simulink model "GNC_exp"  (R2018a)
settings: Solver=FixedStepAuto  StartTime=0.0  StopTime=50  FixedStep=0.05  MaxStep=0.5  MinStep=0.3  RelTol=10  AbsTol=10
values from neighbouring files (symbols this model uses):
  flightplan = [3.3,0,height,deg2rad(0) ... (first row only)    [initialize_exp.m]
  g = 9.81    [initialize_exp.m]
  HFOV = VFOV*resolution(1)/resolution(2)    [initialize_exp.m]
  max_rot_Z = (13)*pi/180    (= 0.226892802759)    [initialize_exp.m]
  max_theta_X = 8*pi/180    (= 0.13962634016)    [initialize_exp.m]
  max_theta_Y = 8*pi/180    (= 0.13962634016)    [initialize_exp.m]
  max_v_Z = 1*max_vel    (= 0.5)    [initialize_exp.m]
  max_vel = 0.5    [initialize_exp.m]
  spline_init = [P0;P1;P2;P3]    [initialize_exp.m]
  two_std_dev_init = [1,1,0.3,deg2rad(15)]    [initialize_exp.m]
  two_std_dev_thres = 0.2    [initialize_exp.m]
  VFOV = 1.05    [initialize_exp.m]
undefined symbols (not defined in the file or in its folder): eul, pos, vel
libraries: sharedtransform x3, aerolibutil x2, simulink x1
(part 1 of 2)
settings Model: EnablePacing=on  Creator=vinni  LastModifiedBy=lenny
settings SolverCC: MaxConsecutiveMinStep=99999  ShapePreserveControl=EnableAll  ZeroCrossAlgorithm=Adaptive
settings DebuggingCC: WriteAfterWriteMsg=EnableAllAsError  AlgebraicLoopMsg=error  IntegerOverflowMsg=error  ParameterUnderflowMsg=error  UniqueDataStoreMsg=error  NonBusSignalsTreatedAsBus=error  IntegerSaturationMsg=error
settings HardwareCC: ProdBitPerLong=64  ProdHWDeviceType=Intel->x86-64 (Linux 64)

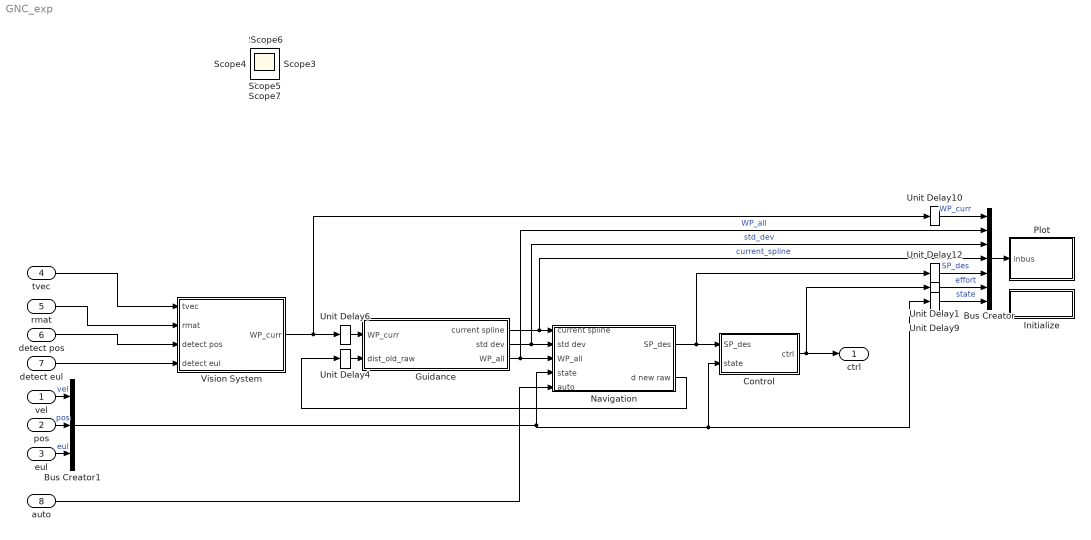
== system GNC_exp ==
  vel : Inport
  pos : Inport  Port=2
  eul : Inport  Port=3
  tvec : Inport  Port=4  PortDimensions=[3,1]
  rmat : Inport  Port=5  PortDimensions=[3,3]
  detect pos : Inport  Port=6  PortDimensions=[3,1]
  detect eul : Inport  Port=7  PortDimensions=[3,1]
  auto : Inport  Port=8
  Bus Creator : BusCreator  Inputs=7  OutDataTypeStr=Bus: PlotBus  NonVirtualBus=on
  Bus Creator1 : BusCreator  Inputs=vel,pos,eul
  Control : Subsystem
  Guidance : Subsystem
  Initialize : Subsystem  TreatAsAtomicUnit=on
  Navigation : Subsystem
  Plot : MATLAB Function  TreatAsAtomicUnit=on
  Unit Delay{1,4,6,9..10,12} (6 alike) : UnitDelay  SampleTime=-1
  Vision System : Subsystem
  ctrl : Outport
  Scope{,1..7} (8 alike) : Scope
  wires:
  Vision System/1(WP_curr) -> Unit Delay10/1, Unit Delay6/1
  Control/1(ctrl) -> Unit Delay1/1, ctrl/1
  Unit Delay6/1 -> Guidance/1(WP_curr)
  Unit Delay4/1 -> Guidance/2(dist_old_raw)
  Navigation/1(SP_des) -> Unit Delay12/1, Control/1(SP_des)
  Navigation/2(d new raw) -> Unit Delay4/1
  Bus Creator1/1 -> Control/2(state), Unit Delay9/1, Navigation/4(state)
  Bus Creator/1 -> Plot/1(inbus)
  Guidance/3(WP_all) -> Navigation/3(WP_all), Bus Creator/2  "WP_all"
  Guidance/2(std dev) -> Navigation/2(std dev), Bus Creator/3  "std_dev"
  Unit Delay9/1 -> Bus Creator/7  "state"
  Unit Delay10/1 -> Bus Creator/1  "WP_curr"
  Unit Delay12/1 -> Bus Creator/5  "SP_des"
  Guidance/1(current spline) -> Navigation/1(current spline), Bus Creator/4  "current_spline"
  Unit Delay1/1 -> Bus Creator/6  "effort"
  pos/1 -> Bus Creator1/2  "pos"
  auto/1 -> Navigation/5(auto)
  eul/1 -> Bus Creator1/3  "eul"
  vel/1 -> Bus Creator1/1  "vel"
  tvec/1 -> Vision System/1(tvec)
  detect eul/1 -> Vision System/4(detect eul)
  rmat/1 -> Vision System/2(rmat)
  detect pos/1 -> Vision System/3(detect pos)

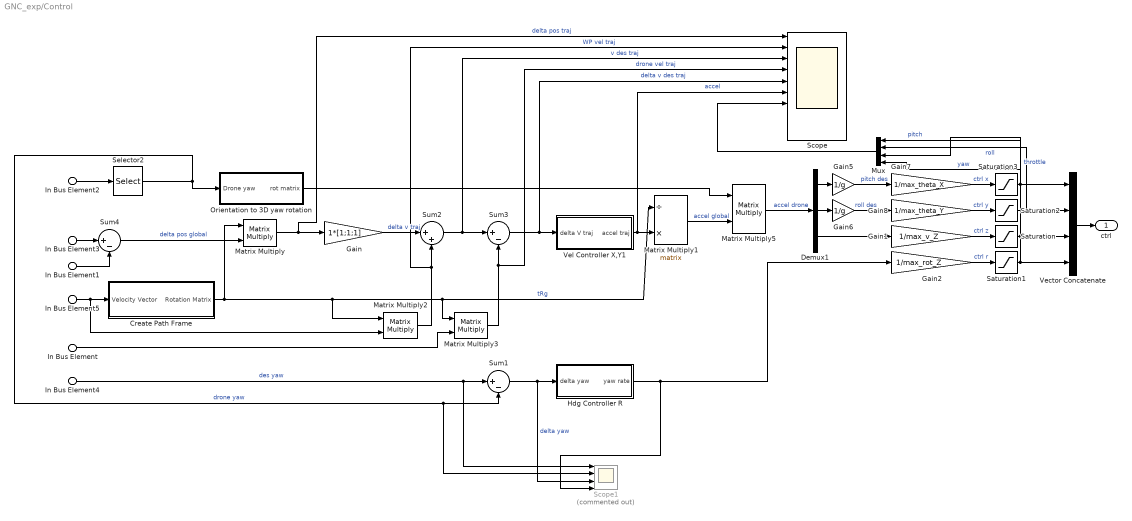
== system GNC_exp/Control ==
  In Bus Element5 : Inport  PortName=SP_des  Element=vel
  In Bus Element3 : Inport  PortName=SP_des  Element=pos
  In Bus Element4 : Inport  PortName=SP_des  Element=yaw
  In Bus Element : Inport  Port=2  PortName=state  Element=vel
  In Bus Element1 : Inport  Port=2  PortName=state  Element=pos
  In Bus Element2 : Inport  Port=2  PortName=state  Element=eul
  Create Path Frame : Subsystem
  Demux1 : Demux  Outputs=3
  Gain : Gain  Gain=1*[1;1;1]
  Gain1 : Gain  Gain=1/max_v_Z
  Gain2 : Gain  Gain=1/max_rot_Z
  Gain5 : Gain  Gain=1/g
  Gain6 : Gain  Gain=1/g
  Gain7 : Gain  Gain=1/max_theta_X
  Gain8 : Gain  Gain=1/max_theta_Y
  Hdg Controller R : Subsystem
  Matrix Multiply{,2..3,5} (4 alike) : Product  Inputs=**  Multiplication=Matrix(*)
  Matrix Multiply1 : Product  Inputs=/*  Multiplication=Matrix(*)
  Mux : Mux
  Orientation to 3D yaw rotation : Subsystem
  Saturation{,1..3} (4 alike) : Saturate  UpperLimit=1  LowerLimit=-1
  Scope : Scope  NumInputPorts=10
  Scope1 : Scope  Commented=on  NumInputPorts=4
  Selector2 : Selector  IndexMode=Zero-based  InputPortWidth=3  IndexOptions=Index vector (dialog)  Indices=2  OutputSizes=1
  Sum1 : Sum  Inputs=|+-
  Sum2 : Sum  Inputs=|++
  Sum3 : Sum  Inputs=|+-
  Sum4 : Sum  Inputs=|+-
  Vector Concatenate : Concatenate  NumInputs=4
  Vel Controller X,Y1 : Subsystem
  ctrl : Outport
  wires:
  Saturation1/1 -> Vector Concatenate/4, Mux/4  "yaw"
  Saturation3/1 -> Vector Concatenate/1, Mux/1  "pitch"
  Saturation2/1 -> Vector Concatenate/2, Mux/2  "roll"
  Saturation/1 -> Vector Concatenate/3, Mux/3  "throttle"
  In Bus Element4/1 -> Scope1/1, Sum1/1  "des yaw"
  In Bus Element3/1 -> Sum4/1
  In Bus Element5/1 -> Matrix Multiply2/2, Create Path Frame/1(Velocity Vector)
  Selector2/1 -> Scope1/2, Sum1/2, Orientation to 3D yaw rotation/1(Drone yaw)  "drone yaw"
  Gain7/1 -> Saturation3/1  "ctrl x"
  Demux1/3 -> Gain1/1
  Hdg Controller R/1(yaw rate) -> Scope1/4, Gain2/1
  Demux1/2 -> Gain6/1
  Mux/1 -> Scope/7
  Gain6/1 -> Gain8/1  "roll des"
  Sum3/1 -> Scope/5, Vel Controller X,Y1/1(delta V traj)  "delta v des traj"
  Matrix Multiply2/1 -> Scope/2, Sum2/2  "WP vel traj"
  Sum4/1 -> Matrix Multiply/2  "delta pos global"
  Matrix Multiply3/1 -> Scope/4, Sum3/2  "drone vel traj"
  Demux1/1 -> Gain5/1
  Gain1/1 -> Saturation/1  "ctrl z"
  Matrix Multiply/1 -> Scope/1, Gain/1  "delta pos traj"
  Gain5/1 -> Gain7/1  "pitch des"
  Vel Controller X,Y1/1(accel traj) -> Scope/6, Matrix Multiply1/2  "accel"
  Matrix Multiply5/1 -> Demux1/1  "accel drone"
  Orientation to 3D yaw rotation/1(rot matrix) -> Matrix Multiply5/1
  Gain8/1 -> Saturation2/1  "ctrl y"
  In Bus Element1/1 -> Sum4/2
  Create Path Frame/1(Rotation Matrix) -> Matrix Multiply/1, Matrix Multiply2/1, Matrix Multiply1/1, Matrix Multiply3/1  "tRg"
  Gain2/1 -> Saturation1/1  "ctrl r"
  In Bus Element/1 -> Matrix Multiply3/2
  Gain/1 -> Sum2/1  "delta v traj"
  Sum2/1 -> Scope/3, Sum3/1  "v des traj"
  Matrix Multiply1/1 -> Matrix Multiply5/2  "accel global"
  Sum1/1 -> Scope1/3, Hdg Controller R/1(delta yaw)  "delta yaw"
  In Bus Element2/1 -> Selector2/1
  Vector Concatenate/1 -> ctrl/1

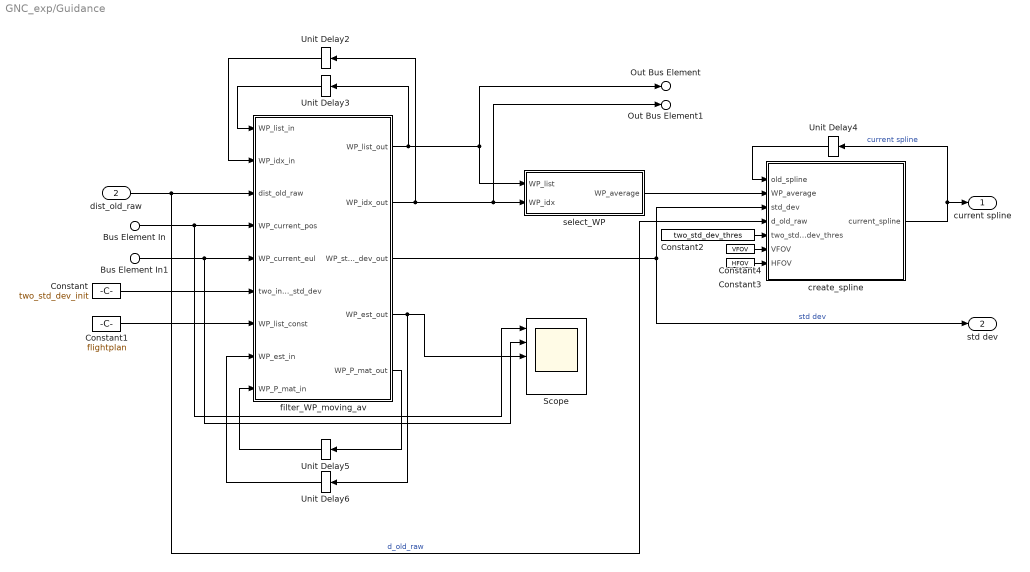
== system GNC_exp/Guidance ==
  Bus Element In1 : Inport  PortName=WP_curr  Element=eul
  Bus Element In : Inport  PortName=WP_curr  Element=pos
  dist_old_raw : Inport  Port=2
  Constant : Constant  Value=two_std_dev_init
  Constant1 : Constant  Value=flightplan
  Constant2 : Constant  Value=two_std_dev_thres
  Constant3 : Constant  Value=HFOV
  Constant4 : Constant  Value=VFOV
  Scope : Scope  NumInputPorts=5
  Unit Delay2 : UnitDelay  SampleTime=-1
  Unit Delay3 : UnitDelay  InitialCondition=flightplan  SampleTime=-1
  Unit Delay4 : UnitDelay  InitialCondition=spline_init  SampleTime=-1
  Unit Delay5 : UnitDelay  InitialCondition=ones(4,4)  SampleTime=-1
  Unit Delay6 : UnitDelay  InitialCondition=ones(1,4)  SampleTime=-1
  create_spline : MATLAB Function  TreatAsAtomicUnit=on
  filter_WP_moving_av : MATLAB Function  TreatAsAtomicUnit=on
  select_WP : MATLAB Function  TreatAsAtomicUnit=on
  current spline : Outport
  std dev : Outport  Port=2
  Out Bus Element : Outport  Port=3  PortName=WP_all  Element=list
  Out Bus Element1 : Outport  Port=3  PortName=WP_all  Element=idx
  wires:
  Bus Element In1/1 -> Scope/2, filter_WP_moving_av/5(WP_current_eul)
  create_spline/1(current_spline) -> Unit Delay4/1, current spline/1  "current spline"
  Bus Element In/1 -> Scope/1, filter_WP_moving_av/4(WP_current_pos)
  select_WP/1(WP_average) -> create_spline/2(WP_average)
  Unit Delay3/1 -> filter_WP_moving_av/1(WP_list_in)
  Unit Delay2/1 -> filter_WP_moving_av/2(WP_idx_in)
  Constant/1 -> filter_WP_moving_av/6(two_init_std_dev)
  filter_WP_moving_av/3(WP_std_dev_out) -> std dev/1, create_spline/3(std_dev)  "std dev"
  filter_WP_moving_av/2(WP_idx_out) -> Out Bus Element1/1, select_WP/2(WP_idx), Unit Delay2/1
  filter_WP_moving_av/1(WP_list_out) -> select_WP/1(WP_list), Out Bus Element/1, Unit Delay3/1
  dist_old_raw/1 -> create_spline/4(d_old_raw), filter_WP_moving_av/3(dist_old_raw)  "d_old_raw"
  Unit Delay4/1 -> create_spline/1(old_spline)
  filter_WP_moving_av/4(WP_est_out) -> Unit Delay6/1, Scope/3
  filter_WP_moving_av/5(WP_P_mat_out) -> Unit Delay5/1
  Unit Delay5/1 -> filter_WP_moving_av/9(WP_P_mat_in)
  Unit Delay6/1 -> filter_WP_moving_av/8(WP_est_in)
  Constant1/1 -> filter_WP_moving_av/7(WP_list_const)
  Constant2/1 -> create_spline/5(two_std_dev_thres)
  Constant3/1 -> create_spline/7(HFOV)
  Constant4/1 -> create_spline/6(VFOV)

== system GNC_exp/Initialize ==
  Event Listener : EventListener  DisableCoverage=on  EventName=reset
  reset_plot : MATLAB Function  TreatAsAtomicUnit=on

== system GNC_exp/Navigation ==
  current spline : Inport
  std dev : Inport  Port=2
  In Bus Element : Inport  Port=3  PortName=WP_all  Element=list
  In Bus Element3 : Inport  Port=3  PortName=WP_all  Element=idx
  In Bus Element1 : Inport  Port=4  PortName=state  Element=pos
  auto : Inport  Port=5
  Constant : Constant  Value=two_std_dev_thres
  Scope : Scope  Commented=on  NumInputPorts=5
  Terminator : Terminator
  calc v : Subsystem
  calculate desired : Subsystem
  get WPts : Subsystem
  select d : MATLAB Function  TreatAsAtomicUnit=on
  set position : Subsystem
  Bus Element Out : Outport  PortName=SP_des  Element=pos
  Bus Element Out1 : Outport  PortName=SP_des  Element=vel
  Bus Element Out2 : Outport  PortName=SP_des  Element=yaw
  d new raw : Outport  Port=2
  wires:
  calculate desired/2(WP vel des) -> Bus Element Out1/1
  current spline/1 -> calc v/1(current spline), calculate desired/2(current spline), set position/1(current spline)
  calculate desired/1(yaw) -> Bus Element Out2/1
  In Bus Element1/1 -> calculate desired/5(drone current pos), calc v/3(drone current pos)
  set position/2(d new raw) -> d new raw/1
  get WPts/3(WP next) -> calculate desired/7(WP next)
  get WPts/2(WP this) -> calc v/4(WP this), calculate desired/6(WP this)
  std dev/1 -> select d/2(std_dev), calculate desired/1(std dev), calc v/2(std dev)
  set position/1(d old1) -> select d/1("d_old "), Scope/4, calculate desired/3(d)
  calculate desired/3(pos) -> calc v/5(drone desired pos), Bus Element Out/1
  calc v/1(velocity) -> Scope/2, calculate desired/4(vel), set position/2(velocity)
  In Bus Element/1 -> get WPts/1(list)
  In Bus Element3/1 -> get WPts/2(idx)
  select d/1(d_old) -> set position/3(d old), calc v/6(d)
  get WPts/1(WP last) -> Terminator/1
  auto/1 -> set position/4(auto)
  Constant/1 -> select d/3(two_std_dev_thres)

== system GNC_exp/Vision System ==
  tvec : Inport
  rmat : Inport  Port=2
  detect pos : Inport  Port=3
  detect eul : Inport  Port=4
  gate_global : MATLAB Function  TreatAsAtomicUnit=on
  Bus Element Out : Outport  PortName=WP_curr  Element=pos
  Bus Element Out1 : Outport  PortName=WP_curr  Element=eul
  wires:
  tvec/1 -> gate_global/1(tVec)  "original image"
  gate_global/2(gate_eul_global) -> Bus Element Out1/1
  gate_global/1(gate_pos_global) -> Bus Element Out/1
  rmat/1 -> gate_global/2(rMat)
  detect pos/1 -> gate_global/3(drone_pos)
  detect eul/1 -> gate_global/4(drone_ori)

== system GNC_exp/Control/Create Path Frame ==
  Velocity Vector : Inport
  Invert 3x3 Matrix : aerolibutil/Invert  3x3 Matrix
  Make X Vector : Subsystem
  Make Y Vector : Subsystem
  Make Z Vector : Subsystem
  Matrix Concatenate : Concatenate  NumInputs=3  Mode=Multidimensional array  ConcatenateDimension=2
  Rotation Matrix : Outport
  wires:
  Velocity Vector/1 -> Make Z Vector/1(Velocity Vector), Make X Vector/1(Velocity Vector), Make Y Vector/1(Velocity Vector)
  Make Y Vector/1(Y Vector) -> Matrix Concatenate/2
  Make X Vector/1(X Vector) -> Matrix Concatenate/1
  Make Z Vector/1(Z Vector) -> Matrix Concatenate/3
  Matrix Concatenate/1 -> Invert 3x3 Matrix/1
  Invert 3x3 Matrix/1 -> Rotation Matrix/1

== system GNC_exp/Control/Hdg Controller R ==
  delta yaw : Inport
  Atan2 : Trigonometry  Operator=atan2
  Cos : Trigonometry  Operator=sincos
  Gain : Gain  Gain=0.1
  PID Controller 0.075 : simulink/Continuous/PID Controller  Controller=PID  TimeDomain=Continuous-time  SampleTime=-1  IntegratorMethod=Forward Euler  FilterMethod=Forward Euler  Form=Parallel  UseFilter=on  ControllerParametersSource=internal  P=0.1  I=0  D=0  N=100  InitialConditionSource=internal  InitialConditionForIntegrator=0  InitialConditionForFilter=0  ExternalReset=none  LimitOutput=off  UpperSaturationLimit=inf  LowerSaturationLimit=-inf  LinearizeAsGain=on  AntiWindupMode=none  Kb=1  TrackingMode=off  Kt=1  PParamMin=[]  PParamMax=[]  IParamMin=[]  IParamMax=[]  DParamMin=[]  DParamMax=[]  NParamMin=[]  NParamMax=[]  KbParamMin=[]  KbParamMax=[]  KtParamMin=[]  KtParamMax=[]  POutMin=[]  POutMax=[]  IOutMin=[]  IOutMax=[]  DOutMin=[]  DOutMax=[]  NOutMin=[]  NOutMax=[]  KbOutMin=[]  KbOutMax=[]  KtOutMin=[]  KtOutMax=[]  IntegratorOutMin=[]  IntegratorOutMax=[]  FilterOutMin=[]  FilterOutMax=[]  SumOutMin=[]  SumOutMax=[]  SumI1OutMin=[]  SumI1OutMax=[]  SumI2OutMin=[]  SumI2OutMax=[]  SumI3OutMin=[]  SumI3OutMax=[]  SumDOutMin=[]  SumDOutMax=[]  SaturationOutMin=[]  SaturationOutMax=[]  IntegratorContinuousStateAttributes=''  IntegratorStateMustResolveToSignalObject=off  IntegratorRTWStateStorageClass=Auto  FilterContinuousStateAttributes=''  FilterStateMustResolveToSignalObject=off  FilterRTWStateStorageClass=Auto  DifferentiatorICPrevScaledInput=0  DifferentiatorOutMin=[]  DifferentiatorOutMax=[]  FilterDiffOutCoefMin=[]  FilterDiffOutCoefMax=[]  SumDenOutMin=[]  SumDenOutMax=[]  SumNumOutMin=[]  SumNumOutMax=[]  ReciprocalOutMin=[]  ReciprocalOutMax=[]  DivideOutMin=[]  DivideOutMax=[]  TunerSelectOption=Transfer Function Based (PID Tuner App)
  yaw rate : Outport
  wires:
  delta yaw/1 -> Cos/1  "delta yaw"
  Cos/1 -> Atan2/1
  Gain/1 -> yaw rate/1  "yaw rate"
  Atan2/1 -> Gain/1  "d yaw"
  Cos/2 -> Atan2/2

== system GNC_exp/Control/Orientation to 3D yaw rotation ==
  note: eul2rotm
  Drone yaw : Inport
  Constant1 : Constant  Value=0
  Rotation Angles to Direction Cosine Matrix : sharedtransform/Rotation Angles to Direction Cosine Matrix  rotationOrder=ZYX  aMode=aMode
      settings: SourceProductBaseCode=AE
  Vector Concatenate : Concatenate  NumInputs=3
  rot matrix : Outport
  wires:
  Constant1/1 -> Vector Concatenate/2, Vector Concatenate/3
  Vector Concatenate/1 -> Rotation Angles to Direction Cosine Matrix/1
  Drone yaw/1 -> Vector Concatenate/1  "yaw"
  Rotation Angles to Direction Cosine Matrix/1 -> rot matrix/1  "rot matrix"

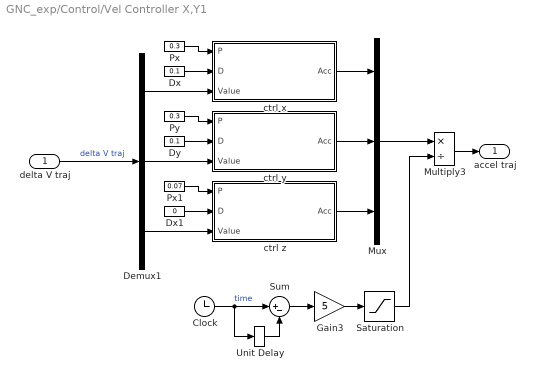
== system GNC_exp/Control/Vel Controller X,Y1 ==
  delta V traj : Inport
  Clock : Clock
  Demux1 : Demux  Outputs=3
  Dx : Constant  Value=0.1
  Dx1 : Constant  Value=0
  Dy : Constant  Value=0.1
  Gain3 : Gain  Gain=5
  Multiply3 : Product  Inputs=*/
  Mux : Mux  Inputs=3
  Px : Constant  Value=0.3
  Px1 : Constant  Value=0.07
  Py : Constant  Value=0.3
  Saturation : Saturate  UpperLimit=100  LowerLimit=0.00001
  Sum : Sum  Inputs=|+-
  Unit Delay : UnitDelay  SampleTime=-1
  ctrl x : Subsystem
  ctrl y : Subsystem
  ctrl z : Subsystem
  accel traj : Outport
  wires:
  delta V traj/1 -> Demux1/1  "delta V traj"
  Mux/1 -> Multiply3/1
  Clock/1 -> Unit Delay/1, Sum/1  "time"
  Unit Delay/1 -> Sum/2
  ctrl z/1(Acc) -> Mux/3
  Sum/1 -> Gain3/1
  Multiply3/1 -> accel traj/1
  Demux1/1 -> ctrl x/3(Value)
  ctrl x/1(Acc) -> Mux/1
  Px/1 -> ctrl x/1(P)
  Dx/1 -> ctrl x/2(D)
  Dy/1 -> ctrl y/2(D)
  Py/1 -> ctrl y/1(P)
  Demux1/2 -> ctrl y/3(Value)
  ctrl y/1(Acc) -> Mux/2
  Saturation/1 -> Multiply3/2
  Gain3/1 -> Saturation/1
  Dx1/1 -> ctrl z/2(D)
  Px1/1 -> ctrl z/1(P)
  Demux1/3 -> ctrl z/3(Value)

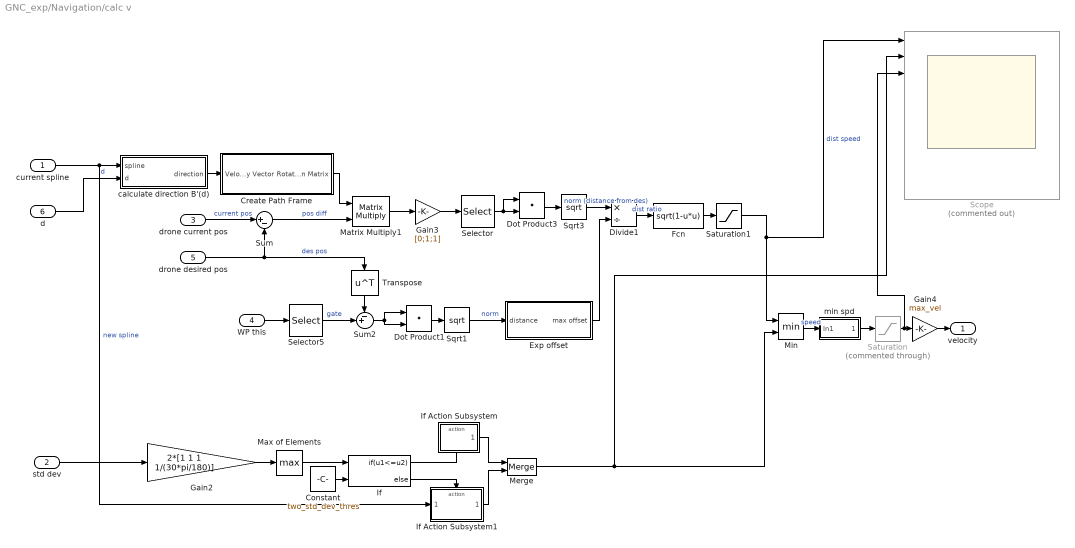
== system GNC_exp/Navigation/calc v ==
  current spline : Inport
  std dev : Inport  Port=2
  drone current pos : Inport  Port=3
  WP this : Inport  Port=4
  drone desired pos : Inport  Port=5
  d : Inport  Port=6
  Constant : Constant  Value=two_std_dev_thres
  Create Path Frame : Subsystem
  Divide1 : Product  Inputs=*/
  Dot Product1 : DotProduct  InputSameDT=on  OutDataTypeStr=Inherit: Inherit via internal rule
  Dot Product3 : DotProduct  InputSameDT=on  OutDataTypeStr=Inherit: Inherit via internal rule
  Exp offset : Subsystem
  Fcn : Fcn  Expr=sqrt(1-u*u)
  Gain2 : Gain  Gain=2*[1 1 1 1/(30*pi/180)]
  Gain3 : Gain  Gain=[0;1;1]
  Gain4 : Gain  Gain=max_vel
  If : If  NumInputs=2  IfExpression=u1<=u2
  If Action Subsystem : Subsystem  TreatAsAtomicUnit=on
  If Action Subsystem1 : Subsystem  TreatAsAtomicUnit=on
  Matrix Multiply1 : Product  Inputs=**  Multiplication=Matrix(*)
  Max of Elements : MinMax  Function=max
  Merge : Merge
  Min : MinMax  Inputs=2
  Saturation : Saturate  Commented=through  UpperLimit=1.01  LowerLimit=0.99
  Saturation1 : Saturate  UpperLimit=1  LowerLimit=0
  Scope : Scope  Commented=on  NumInputPorts=10
  Selector : Selector  IndexMode=Zero-based  InputPortWidth=3  IndexOptions=Index vector (dialog)  Indices=[0 1 2]  OutputSizes=1
  Selector5 : Selector  NumberOfDimensions=2  IndexMode=Zero-based  InputPortWidth=4  IndexOptions=Select all,Index vector (dialog)  Indices=[1 2 3],[0 1 2]  OutputSizes=1,1
  Sqrt1 : Sqrt  SaturateOnIntegerOverflow=on
  Sqrt3 : Sqrt  SaturateOnIntegerOverflow=on
  Sum : Sum  Inputs=|+-
  Sum2 : Sum  Inputs=-+|
  Transpose : Math  Operator=transpose  SaturateOnIntegerOverflow=on
  calculate direction B'(d) : Subsystem
  min spd : Subsystem
  velocity : Outport
  wires:
  If Action Subsystem1/1(red vel) -> Merge/2
  If Action Subsystem/1(1) -> Merge/1
  If/1 -> If Action Subsystem/Action
  std dev/1 -> Gain2/1
  If/2 -> If Action Subsystem1/Action
  Gain2/1 -> Max of Elements/1
  Max of Elements/1 -> If/1
  Create Path Frame/1(Rotation Matrix) -> Matrix Multiply1/1
  Sum2/1 -> Dot Product1/1, Dot Product1/2
  Min/1 -> min spd/1(In1)  "speed"
  Fcn/1 -> Saturation1/1
  Saturation/1 -> Scope/3, Gain4/1
  Dot Product3/1 -> Sqrt3/1
  Selector5/1 -> Sum2/2  "gate"
  calculate direction B'(d)/1(direction) -> Create Path Frame/1(Velocity Vector)
  Divide1/1 -> Fcn/1  "dist ratio"
  Selector/1 -> Dot Product3/1, Dot Product3/2
  d/1 -> calculate direction B'(d)/2(d)  "d"
  Sum/1 -> Matrix Multiply1/2  "pos diff"
  Merge/1 -> Scope/2, Min/2
  Sqrt1/1 -> Exp offset/1(distance)  "norm"
  Dot Product1/1 -> Sqrt1/1
  drone desired pos/1 -> Transpose/1, Sum/2  "des pos"
  Saturation1/1 -> Scope/1, Min/1  "dist speed"
  Exp offset/1(max offset) -> Divide1/2
  Gain4/1 -> velocity/1
  Sqrt3/1 -> Divide1/1  "norm (distance from des)"
  drone current pos/1 -> Sum/1  "current pos"
  Transpose/1 -> Sum2/1
  min spd/1(Out1) -> Saturation/1
  Matrix Multiply1/1 -> Gain3/1
  current spline/1 -> If Action Subsystem1/1(spline), calculate direction B'(d)/1(spline)  "new spline"
  WP this/1 -> Selector5/1
  Constant/1 -> If/2
  Gain3/1 -> Selector/1

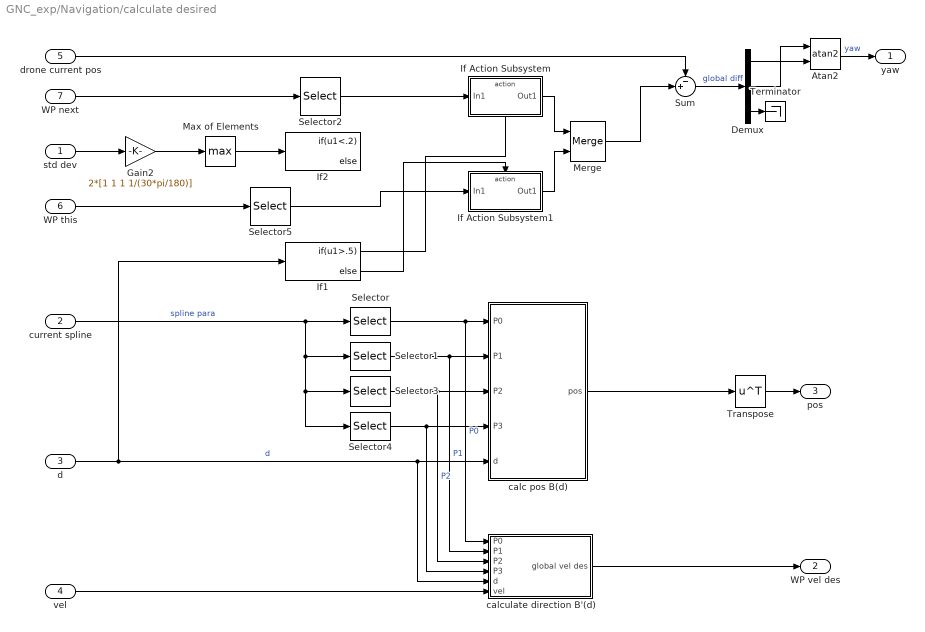
== system GNC_exp/Navigation/calculate desired ==
  std dev : Inport
  current spline : Inport  Port=2
  d : Inport  Port=3
  vel : Inport  Port=4
  drone current pos : Inport  Port=5
  WP this : Inport  Port=6
  WP next : Inport  Port=7
  Atan2 : Trigonometry  Operator=atan2
  Demux : Demux  Outputs=3
  Gain2 : Gain  Gain=2*[1 1 1 1/(30*pi/180)]
  If Action Subsystem : Subsystem  TreatAsAtomicUnit=on
  If Action Subsystem1 : Subsystem  TreatAsAtomicUnit=on
  If1 : If  IfExpression=u1>.5
  If2 : If  IfExpression=u1<.2
  Max of Elements : MinMax  Function=max
  Merge : Merge
  Selector : Selector  NumberOfDimensions=2  IndexMode=Zero-based  InputPortWidth=3  IndexOptions=Index vector (dialog),Select all  Indices=0,[0 1 2]  OutputSizes=1,1
  Selector1 : Selector  NumberOfDimensions=2  IndexMode=Zero-based  InputPortWidth=3  IndexOptions=Index vector (dialog),Select all  Indices=1,[0 1 2]  OutputSizes=1,1
  Selector2 : Selector  NumberOfDimensions=2  IndexMode=Zero-based  InputPortWidth=4  IndexOptions=Select all,Index vector (dialog)  Indices=[1 2 3],[0 1 2]  OutputSizes=1,1
  Selector3 : Selector  NumberOfDimensions=2  IndexMode=Zero-based  InputPortWidth=3  IndexOptions=Index vector (dialog),Select all  Indices=2,[0 1 2]  OutputSizes=1,1
  Selector4 : Selector  NumberOfDimensions=2  IndexMode=Zero-based  InputPortWidth=3  IndexOptions=Index vector (dialog),Select all  Indices=3,[0 1 2]  OutputSizes=1,1
  Selector5 : Selector  NumberOfDimensions=2  IndexMode=Zero-based  InputPortWidth=4  IndexOptions=Select all,Index vector (dialog)  Indices=[1 2 3],[0 1 2]  OutputSizes=1,1
  Sum : Sum  Inputs=-+|
  Terminator : Terminator
  Transpose : Math  Operator=transpose  SaturateOnIntegerOverflow=on
  calc pos B(d) : Subsystem
  calculate direction B'(d) : Subsystem
  yaw : Outport
  WP vel des : Outport  Port=2
  pos : Outport  Port=3
  wires:
  current spline/1 -> Selector4/1, Selector3/1, Selector1/1, Selector/1  "spline para"
  Selector/1 -> calculate direction B'(d)/1(P0), calc pos B(d)/1(P0)  "P0"
  Selector1/1 -> calculate direction B'(d)/2(P1), calc pos B(d)/2(P1)  "P1"
  Selector3/1 -> calculate direction B'(d)/3(P2), calc pos B(d)/3(P2)  "P2"
  d/1 -> If1/1, calc pos B(d)/5(d), calculate direction B'(d)/5(d)  "d"
  calc pos B(d)/1(pos) -> Transpose/1
  Sum/1 -> Demux/1  "global diff"
  Demux/2 -> Atan2/1
  Demux/1 -> Atan2/2
  Demux/3 -> Terminator/1
  Atan2/1 -> yaw/1  "yaw"
  vel/1 -> calculate direction B'(d)/6(vel)
  calculate direction B'(d)/1(global vel des) -> WP vel des/1
  Transpose/1 -> pos/1
  drone current pos/1 -> Sum/1
  WP next/1 -> Selector2/1
  If Action Subsystem/1(Out1) -> Merge/1
  If Action Subsystem1/1(Out1) -> Merge/2
  WP this/1 -> Selector5/1
  Selector2/1 -> If Action Subsystem/1(In1)
  Selector4/1 -> calc pos B(d)/4(P3), calculate direction B'(d)/4(P3)
  Merge/1 -> Sum/2
  std dev/1 -> Gain2/1
  Gain2/1 -> Max of Elements/1
  Max of Elements/1 -> If2/1
  If1/1 -> If Action Subsystem/Action
  Selector5/1 -> If Action Subsystem1/1(In1)
  If1/2 -> If Action Subsystem1/Action

== system GNC_exp/Navigation/get WPts ==
  list : Inport
  idx : Inport  Port=2
  Fcn : Fcn  Expr=u-1
  Fcn1 : Fcn  Expr=u+1
  Mod : Math  Operator=mod  SaturateOnIntegerOverflow=on
  Mod1 : Math  Operator=mod  SaturateOnIntegerOverflow=on
  Mod2 : Math  Operator=mod  SaturateOnIntegerOverflow=on
  Probe Dimension : Probe  ProbeWidth=off  ProbeSampleTime=off  ProbeComplexSignal=off  ProbeSignalDimensions=on
  Selector : Selector  InputPortWidth=2  IndexOptions=Index vector (dialog)  Indices=1  OutputSizes=1
  Selector1 : Selector  NumberOfDimensions=2  IndexMode=Zero-based  InputPortWidth=3  IndexOptions=Index vector (port),Select all  Indices=[1 3],1  OutputSizes=1,1
  Selector2 : Selector  NumberOfDimensions=2  IndexMode=Zero-based  InputPortWidth=3  IndexOptions=Index vector (port),Select all  Indices=[1 3],1  OutputSizes=1,1
  Selector3 : Selector  NumberOfDimensions=2  IndexMode=Zero-based  InputPortWidth=3  IndexOptions=Index vector (port),Select all  Indices=[1 3],1  OutputSizes=1,1
  WP last : Outport
  WP this : Outport  Port=2
  WP next : Outport  Port=3
  wires:
  list/1 -> Selector3/1, Selector2/1, Selector1/1, Probe Dimension/1
  idx/1 -> Fcn/1, Mod1/1, Fcn1/1
  Fcn/1 -> Mod/1
  Mod/1 -> Selector1/2
  Fcn1/1 -> Mod2/1
  Probe Dimension/1 -> Selector/1
  Selector/1 -> Mod2/2, Mod1/2, Mod/2
  Mod1/1 -> Selector2/2
  Mod2/1 -> Selector3/2
  Selector1/1 -> WP last/1
  Selector2/1 -> WP this/1
  Selector3/1 -> WP next/1

== system GNC_exp/Navigation/set position ==
  current spline : Inport
  velocity : Inport  Port=2
  d old : Inport  Port=3
  auto : Inport  Port=4
  Constant2 : Constant
  Mod1 : Math  Operator=mod  SaturateOnIntegerOverflow=on
  Selector10 : Selector  NumberOfDimensions=2  IndexMode=Zero-based  InputPortWidth=3  IndexOptions=Index vector (dialog),Select all  Indices=1,[0 1 2]  OutputSizes=1,1
  Selector11 : Selector  NumberOfDimensions=2  IndexMode=Zero-based  InputPortWidth=3  IndexOptions=Index vector (dialog),Select all  Indices=2,[0 1 2]  OutputSizes=1,1
  Selector12 : Selector  NumberOfDimensions=2  IndexMode=Zero-based  InputPortWidth=3  IndexOptions=Index vector (dialog),Select all  Indices=3,[0 1 2]  OutputSizes=1,1
  Selector7 : Selector  NumberOfDimensions=2  IndexMode=Zero-based  InputPortWidth=3  IndexOptions=Index vector (dialog),Select all  Indices=0,[0 1 2]  OutputSizes=1,1
  Unit Delay2 : UnitDelay  SampleTime=-1
  new d with linearization : Subsystem
  d old1 : Outport
  d new raw : Outport  Port=2
  wires:
  current spline/1 -> Selector7/1, Selector10/1, Selector11/1, Selector12/1  "spline para"
  Selector7/1 -> new d with linearization/3(P0)  "P0"
  Selector10/1 -> new d with linearization/4(P1)  "P1"
  Selector11/1 -> new d with linearization/5(P2)  "P2"
  Selector12/1 -> new d with linearization/6(P3)  "P3"
  d old/1 -> new d with linearization/2(d old)
  velocity/1 -> new d with linearization/1(vel)
  new d with linearization/1(d new same spline) -> d new raw/1, Mod1/1  "d new over"
  Mod1/1 -> Unit Delay2/1
  Constant2/1 -> Mod1/2
  Unit Delay2/1 -> d old1/1
  auto/1 -> new d with linearization/7(auto)

== system GNC_exp/Control/Create Path Frame/Make X Vector ==
  Velocity Vector : Inport
  Make Unit : Subsystem
  X Vector : Outport
  wires:
  Velocity Vector/1 -> Make Unit/1(Vector)
  Make Unit/1(Unit Vector) -> X Vector/1

== system GNC_exp/Control/Create Path Frame/Make Y Vector ==
  Velocity Vector : Inport
  Constant : Constant  Value=0
  Demux : Demux  Outputs=3
  Gain : Gain  Gain=-1
  Make Unit : Subsystem
  Matrix Concatenate : Concatenate  NumInputs=3  Mode=Multidimensional array
  Terminator : Terminator
  Y Vector : Outport
  wires:
  Make Unit/1(Unit Vector) -> Y Vector/1
  Velocity Vector/1 -> Demux/1
  Demux/3 -> Terminator/1
  Demux/2 -> Gain/1
  Gain/1 -> Matrix Concatenate/1
  Demux/1 -> Matrix Concatenate/2
  Constant/1 -> Matrix Concatenate/3
  Matrix Concatenate/1 -> Make Unit/1(Vector)

== system GNC_exp/Control/Create Path Frame/Make Z Vector ==
  Velocity Vector : Inport
  Add : Sum
  Demux : Demux  Outputs=3
  Gain : Gain  Gain=-1
  Gain1 : Gain  Gain=-1
  Make Unit : Subsystem
  Matrix Concatenate : Concatenate  NumInputs=3  Mode=Multidimensional array
  Multiply : Product
  Multiply1 : Product
  Square : Math  Operator=square  SaturateOnIntegerOverflow=on
  Square1 : Math  Operator=square  SaturateOnIntegerOverflow=on
  Z Vector : Outport
  wires:
  Make Unit/1(Unit Vector) -> Z Vector/1
  Velocity Vector/1 -> Demux/1
  Demux/3 -> Multiply/2, Multiply1/2
  Matrix Concatenate/1 -> Make Unit/1(Vector)
  Multiply/1 -> Gain/1
  Gain/1 -> Matrix Concatenate/1
  Demux/1 -> Square/1, Multiply/1
  Multiply1/1 -> Gain1/1
  Gain1/1 -> Matrix Concatenate/2
  Demux/2 -> Square1/1, Multiply1/1
  Add/1 -> Matrix Concatenate/3
  Square/1 -> Add/1
  Square1/1 -> Add/2

== system GNC_exp/Control/Vel Controller X,Y1/ctrl x ==
  P : Inport
  D : Inport  Port=2
  Value : Inport  Port=3
  Add : Sum  Inputs=+++
  Add1 : Sum
  Gain : Gain  Gain=3
  Gain1 : Gain
  Gain2 : Gain  Gain=2
  Gain3 : Gain  Gain=0.1
  Multiply : Product
  Multiply1 : Product
  Sum : Sum  Inputs=-+|
  Sum1 : Sum  Inputs=-+|
  Sum2 : Sum  Inputs=-+|
  Unit Delay1 : UnitDelay  SampleTime=-1
  Unit Delay2 : UnitDelay  SampleTime=-1
  Unit Delay3 : UnitDelay  SampleTime=-1
  Acc : Outport
  wires:
  Unit Delay1/1 -> Sum/1, Unit Delay2/1
  Multiply1/1 -> Add1/2  "P"
  Multiply/1 -> Sum/2, Sum1/2, Sum2/2, Unit Delay1/1
  Gain3/1 -> Add1/1  "D"
  Unit Delay2/1 -> Sum1/1, Unit Delay3/1
  Value/1 -> Multiply1/1, Multiply/2
  Unit Delay3/1 -> Sum2/1
  Add1/1 -> Acc/1
  D/1 -> Multiply/1
  P/1 -> Multiply1/2
  Sum2/1 -> Gain1/1
  Sum1/1 -> Gain2/1
  Sum/1 -> Gain/1
  Gain1/1 -> Add/1
  Gain2/1 -> Add/2
  Gain/1 -> Add/3
  Add/1 -> Gain3/1

== system GNC_exp/Control/Vel Controller X,Y1/ctrl y ==
  P : Inport
  D : Inport  Port=2
  Value : Inport  Port=3
  Add : Sum  Inputs=+++
  Add1 : Sum
  Gain : Gain  Gain=3
  Gain1 : Gain
  Gain2 : Gain  Gain=2
  Gain3 : Gain  Gain=0.1
  Multiply : Product
  Multiply1 : Product
  Sum : Sum  Inputs=-+|
  Sum1 : Sum  Inputs=-+|
  Sum2 : Sum  Inputs=-+|
  Unit Delay1 : UnitDelay  SampleTime=-1
  Unit Delay2 : UnitDelay  SampleTime=-1
  Unit Delay3 : UnitDelay  SampleTime=-1
  Acc : Outport
  wires:
  Unit Delay1/1 -> Sum/1, Unit Delay2/1
  Multiply1/1 -> Add1/2  "P"
  Multiply/1 -> Sum/2, Sum1/2, Sum2/2, Unit Delay1/1
  Gain3/1 -> Add1/1  "D"
  Unit Delay2/1 -> Sum1/1, Unit Delay3/1
  Value/1 -> Multiply1/1, Multiply/2
  Unit Delay3/1 -> Sum2/1
  Add1/1 -> Acc/1
  D/1 -> Multiply/1
  P/1 -> Multiply1/2
  Sum2/1 -> Gain1/1
  Sum1/1 -> Gain2/1
  Sum/1 -> Gain/1
  Gain1/1 -> Add/1
  Gain2/1 -> Add/2
  Gain/1 -> Add/3
  Add/1 -> Gain3/1

== system GNC_exp/Control/Vel Controller X,Y1/ctrl z ==
  P : Inport
  D : Inport  Port=2
  Value : Inport  Port=3
  Add : Sum  Inputs=+++
  Add1 : Sum
  Gain : Gain  Gain=3
  Gain1 : Gain
  Gain2 : Gain  Gain=2
  Gain3 : Gain  Gain=0.1
  Multiply : Product
  Multiply1 : Product
  Sum : Sum  Inputs=-+|
  Sum1 : Sum  Inputs=-+|
  Sum2 : Sum  Inputs=-+|
  Unit Delay1 : UnitDelay  SampleTime=-1
  Unit Delay2 : UnitDelay  SampleTime=-1
  Unit Delay3 : UnitDelay  SampleTime=-1
  Acc : Outport
  wires:
  Unit Delay1/1 -> Sum/1, Unit Delay2/1
  Multiply1/1 -> Add1/2  "P"
  Multiply/1 -> Sum/2, Sum1/2, Sum2/2, Unit Delay1/1
  Gain3/1 -> Add1/1  "D"
  Unit Delay2/1 -> Sum1/1, Unit Delay3/1
  Value/1 -> Multiply1/1, Multiply/2
  Unit Delay3/1 -> Sum2/1
  Add1/1 -> Acc/1
  D/1 -> Multiply/1
  P/1 -> Multiply1/2
  Sum2/1 -> Gain1/1
  Sum1/1 -> Gain2/1
  Sum/1 -> Gain/1
  Gain1/1 -> Add/1
  Gain2/1 -> Add/2
  Gain/1 -> Add/3
  Add/1 -> Gain3/1

== system GNC_exp/Navigation/calc v/Create Path Frame ==
  Velocity Vector : Inport
  Invert 3x3 Matrix : aerolibutil/Invert  3x3 Matrix
  Make X Vector : Subsystem
  Make Y Vector : Subsystem
  Make Z Vector : Subsystem
  Matrix Concatenate : Concatenate  NumInputs=3  Mode=Multidimensional array  ConcatenateDimension=2
  Rotation Matrix : Outport
  wires:
  Velocity Vector/1 -> Make Z Vector/1(Velocity Vector), Make X Vector/1(Velocity Vector), Make Y Vector/1(Velocity Vector)
  Make Y Vector/1(Y Vector) -> Matrix Concatenate/2
  Make X Vector/1(X Vector) -> Matrix Concatenate/1
  Make Z Vector/1(Z Vector) -> Matrix Concatenate/3
  Matrix Concatenate/1 -> Invert 3x3 Matrix/1
  Invert 3x3 Matrix/1 -> Rotation Matrix/1

== system GNC_exp/Navigation/calc v/Exp offset ==
  note: y=s-(s-b) e^{-k(x-d)}
  distance : Inport
  Exp : Math  SaturateOnIntegerOverflow=on
  Gain : Gain  Gain=-1
  Minus : Sum  Inputs=-+
  Multiply : Product
  Multiply1 : Product
  Sum : Sum  Inputs=-+|
  Sum1 : Sum  Inputs=|-+
  b : Constant
  d : Constant  Value=2.5
  k : Constant  Value=-.8
  s : Constant  Value=.1
  max offset : Outport
  wires:
  distance/1 -> Sum/2
  d/1 -> Sum/1
  k/1 -> Gain/1
  Gain/1 -> Multiply/2
  Sum/1 -> Multiply/1
  Multiply/1 -> Exp/1
  b/1 -> Sum1/1
  Exp/1 -> Multiply1/1
  Sum1/1 -> Multiply1/2
  s/1 -> Minus/2, Sum1/2
  Multiply1/1 -> Minus/1
  Minus/1 -> max offset/1

== system GNC_exp/Navigation/calc v/If Action Subsystem ==
  Action Port : ActionPort  ActionType=then
  Constant : Constant
  1 : Outport
  wires:
  Constant/1 -> 1/1

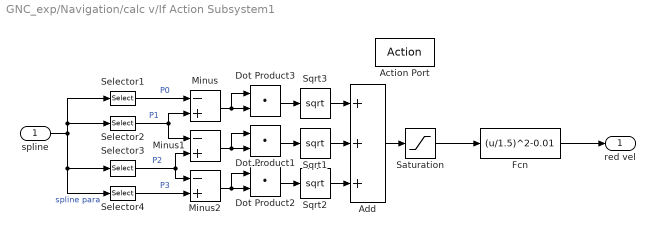
== system GNC_exp/Navigation/calc v/If Action Subsystem1 ==
  spline : Inport
  Action Port : ActionPort  ActionType=else
  Add : Sum  Inputs=+++
  Dot Product1 : DotProduct  InputSameDT=on  OutDataTypeStr=Inherit: Inherit via internal rule
  Dot Product2 : DotProduct  InputSameDT=on  OutDataTypeStr=Inherit: Inherit via internal rule
  Dot Product3 : DotProduct  InputSameDT=on  OutDataTypeStr=Inherit: Inherit via internal rule
  Fcn : Fcn  Expr=(u/1.5)^2-0.01
  Minus : Sum  Inputs=-+
  Minus1 : Sum  Inputs=-+
  Minus2 : Sum  Inputs=-+
  Saturation : Saturate  UpperLimit=1.5  LowerLimit=-1
  Selector1 : Selector  NumberOfDimensions=2  IndexMode=Zero-based  InputPortWidth=3  IndexOptions=Index vector (dialog),Select all  Indices=0,[0 1 2]  OutputSizes=1,1
  Selector2 : Selector  NumberOfDimensions=2  IndexMode=Zero-based  InputPortWidth=3  IndexOptions=Index vector (dialog),Select all  Indices=1,[0 1 2]  OutputSizes=1,1
  Selector3 : Selector  NumberOfDimensions=2  IndexMode=Zero-based  InputPortWidth=3  IndexOptions=Index vector (dialog),Select all  Indices=2,[0 1 2]  OutputSizes=1,1
  Selector4 : Selector  NumberOfDimensions=2  IndexMode=Zero-based  InputPortWidth=3  IndexOptions=Index vector (dialog),Select all  Indices=3,[0 1 2]  OutputSizes=1,1
  Sqrt1 : Sqrt  SaturateOnIntegerOverflow=on
  Sqrt2 : Sqrt  SaturateOnIntegerOverflow=on
  Sqrt3 : Sqrt  SaturateOnIntegerOverflow=on
  red vel : Outport
  wires:
  Saturation/1 -> Fcn/1
  Fcn/1 -> red vel/1
  Selector2/1 -> Minus1/1, Minus/2  "P1"
  Selector3/1 -> Minus2/1, Minus1/2  "P2"
  Selector4/1 -> Minus2/2  "P3"
  spline/1 -> Selector2/1, Selector1/1, Selector4/1, Selector3/1  "spline para"
  Selector1/1 -> Minus/1  "P0"
  Minus/1 -> Dot Product3/1, Dot Product3/2
  Dot Product3/1 -> Sqrt3/1
  Sqrt3/1 -> Add/1
  Minus1/1 -> Dot Product1/1, Dot Product1/2
  Dot Product1/1 -> Sqrt1/1
  Minus2/1 -> Dot Product2/1, Dot Product2/2
  Dot Product2/1 -> Sqrt2/1
  Sqrt1/1 -> Add/2
  Sqrt2/1 -> Add/3
  Add/1 -> Saturation/1

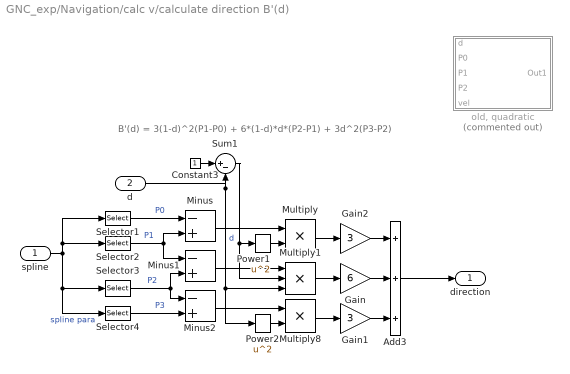
== system GNC_exp/Navigation/calc v/calculate direction B'(d) ==
  note: B'(d) = 3(1-d)^2(P1-P0) + 6*(1-d)*d*(P2-P1) + 3d^2(P3-P2)
  spline : Inport
  d : Inport  Port=2
  Add3 : Sum  Inputs=+++
  Constant3 : Constant
  Gain : Gain  Gain=6
  Gain1 : Gain  Gain=3
  Gain2 : Gain  Gain=3
  Minus : Sum  Inputs=-+
  Minus1 : Sum  Inputs=-+
  Minus2 : Sum  Inputs=-+
  Multiply : Product
  Multiply1 : Product  Inputs=3
  Multiply8 : Product
  Power1 : Math  Operator=square  SaturateOnIntegerOverflow=on
  Power2 : Math  Operator=square  SaturateOnIntegerOverflow=on
  Selector1 : Selector  NumberOfDimensions=2  IndexMode=Zero-based  InputPortWidth=3  IndexOptions=Index vector (dialog),Select all  Indices=0,[0 1 2]  OutputSizes=1,1
  Selector2 : Selector  NumberOfDimensions=2  IndexMode=Zero-based  InputPortWidth=3  IndexOptions=Index vector (dialog),Select all  Indices=1,[0 1 2]  OutputSizes=1,1
  Selector3 : Selector  NumberOfDimensions=2  IndexMode=Zero-based  InputPortWidth=3  IndexOptions=Index vector (dialog),Select all  Indices=2,[0 1 2]  OutputSizes=1,1
  Selector4 : Selector  NumberOfDimensions=2  IndexMode=Zero-based  InputPortWidth=3  IndexOptions=Index vector (dialog),Select all  Indices=3,[0 1 2]  OutputSizes=1,1
  Sum1 : Sum  Inputs=|+-
  "old, quadratic" : Subsystem  Commented=on
  direction : Outport
  wires:
  Sum1/1 -> Multiply1/2, Power1/1
  Minus1/1 -> Multiply1/1
  Minus/1 -> Multiply/1
  Gain/1 -> Add3/2
  Gain1/1 -> Add3/3
  Multiply1/1 -> Gain/1
  Minus2/1 -> Multiply8/1
  Constant3/1 -> Sum1/1
  Multiply/1 -> Gain2/1
  Multiply8/1 -> Gain1/1
  Power2/1 -> Multiply8/2
  Power1/1 -> Multiply/2
  d/1 -> Sum1/2, Power2/1, Multiply1/3  "d"
  Gain2/1 -> Add3/1
  Add3/1 -> direction/1
  Selector1/1 -> Minus/1  "P0"
  Selector3/1 -> Minus2/1, Minus1/2  "P2"
  spline/1 -> Selector2/1, Selector1/1, Selector4/1, Selector3/1  "spline para"
  Selector2/1 -> Minus1/1, Minus/2  "P1"
  Selector4/1 -> Minus2/2  "P3"

== system GNC_exp/Navigation/calc v/min spd ==
  In1 : Inport
  Abs : Abs
  Add : Sum  Inputs=+-
  Constant : Constant  Value=0.01
  Constant1 : Constant  Value=0.5
  Minus : Sum  Inputs=+-
  Multiply : Product
  Saturation : Saturate  UpperLimit=0  LowerLimit=-1
  Scope : Scope  Commented=on  NumInputPorts=7
  Sign : Signum
  Sign1 : Signum
  Sum : Sum  Inputs=|++
  Out1 : Outport
  wires:
  In1/1 -> Scope/1, Add/1, Sign/1, Abs/1
  Abs/1 -> Minus/1
  Constant/1 -> Minus/2
  Minus/1 -> Scope/4, Saturation/1
  Saturation/1 -> Scope/5, Multiply/1
  Sum/1 -> Sign1/1
  Multiply/1 -> Scope/2, Add/2
  Add/1 -> Scope/3, Out1/1
  Constant1/1 -> Sum/2
  Sign1/1 -> Multiply/2
  Sign/1 -> Sum/1

== system GNC_exp/Navigation/calculate desired/If Action Subsystem ==
  In1 : Inport
  Action Port : ActionPort  ActionType=then
  Out1 : Outport
  wires:
  In1/1 -> Out1/1

== system GNC_exp/Navigation/calculate desired/If Action Subsystem1 ==
  In1 : Inport
  Action Port : ActionPort  ActionType=else
  Out1 : Outport
  wires:
  In1/1 -> Out1/1

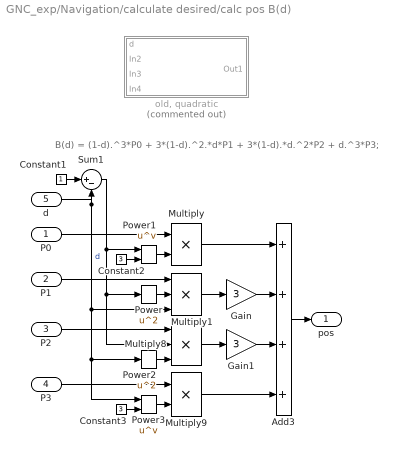
== system GNC_exp/Navigation/calculate desired/calc pos B(d) ==
  note: B(d) = (1-d).^3*P0 + 3*(1-d).^2.*d*P1 + 3*(1-d).*d.^2*P2 + d.^3*P3;
  P0 : Inport
  P1 : Inport  Port=2
  P2 : Inport  Port=3
  P3 : Inport  Port=4
  d : Inport  Port=5
  Add3 : Sum  Inputs=++++
  Constant1 : Constant
  Constant2 : Constant  Value=3
  Constant3 : Constant  Value=3
  Gain : Gain  Gain=3
  Gain1 : Gain  Gain=3
  Multiply : Product
  Multiply1 : Product  Inputs=3
  Multiply8 : Product  Inputs=3
  Multiply9 : Product
  Power : Math  Operator=square  SaturateOnIntegerOverflow=on
  Power1 : Math  Operator=pow  SaturateOnIntegerOverflow=on
  Power2 : Math  Operator=square  SaturateOnIntegerOverflow=on
  Power3 : Math  Operator=pow  SaturateOnIntegerOverflow=on
  Sum1 : Sum  Inputs=|+-
  "old, quadratic" : Subsystem  Commented=on
  pos : Outport
  wires:
  Gain/1 -> Add3/2
  Gain1/1 -> Add3/3
  P1/1 -> Multiply1/1
  P0/1 -> Multiply/1
  P2/1 -> Multiply8/1
  P3/1 -> Multiply9/1
  Multiply/1 -> Add3/1
  Multiply1/1 -> Gain/1
  Multiply8/1 -> Gain1/1
  Multiply9/1 -> Add3/4
  Add3/1 -> pos/1
  Constant1/1 -> Sum1/1
  d/1 -> Sum1/2, Multiply1/3, Power2/1, Power3/1  "d"
  Power/1 -> Multiply1/2
  Power1/1 -> Multiply/2
  Power2/1 -> Multiply8/3
  Power3/1 -> Multiply9/2
  Constant2/1 -> Power1/2
  Constant3/1 -> Power3/2
  Sum1/1 -> Multiply8/2, Power/1, Power1/1

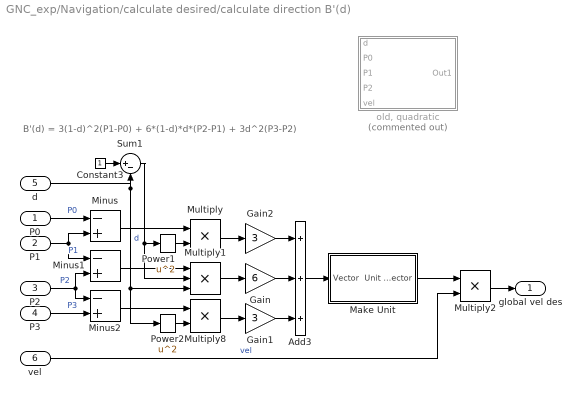
== system GNC_exp/Navigation/calculate desired/calculate direction B'(d) ==
  note: B'(d) = 3(1-d)^2(P1-P0) + 6*(1-d)*d*(P2-P1) + 3d^2(P3-P2)
  P0 : Inport
  P1 : Inport  Port=2
  P2 : Inport  Port=3
  P3 : Inport  Port=4
  d : Inport  Port=5
  vel : Inport  Port=6
  Add3 : Sum  Inputs=+++
  Constant3 : Constant
  Gain : Gain  Gain=6
  Gain1 : Gain  Gain=3
  Gain2 : Gain  Gain=3
  Make Unit : Subsystem
  Minus : Sum  Inputs=-+
  Minus1 : Sum  Inputs=-+
  Minus2 : Sum  Inputs=-+
  Multiply : Product
  Multiply1 : Product  Inputs=3
  Multiply2 : Product
  Multiply8 : Product
  Power1 : Math  Operator=square  SaturateOnIntegerOverflow=on
  Power2 : Math  Operator=square  SaturateOnIntegerOverflow=on
  Sum1 : Sum  Inputs=|+-
  "old, quadratic" : Subsystem  Commented=on
  global vel des : Outport
  wires:
  Sum1/1 -> Multiply1/2, Power1/1
  Minus1/1 -> Multiply1/1
  Minus/1 -> Multiply/1
  Gain/1 -> Add3/2
  Gain1/1 -> Add3/3
  Multiply1/1 -> Gain/1
  Minus2/1 -> Multiply8/1
  Constant3/1 -> Sum1/1
  Multiply/1 -> Gain2/1
  Multiply8/1 -> Gain1/1
  Power2/1 -> Multiply8/2
  Power1/1 -> Multiply/2
  d/1 -> Sum1/2, Power2/1, Multiply1/3  "d"
  Gain2/1 -> Add3/1
  P0/1 -> Minus/1  "P0"
  P1/1 -> Minus/2, Minus1/1  "P1"
  P2/1 -> Minus1/2, Minus2/1  "P2"
  P3/1 -> Minus2/2  "P3"
  Multiply2/1 -> global vel des/1
  Add3/1 -> Make Unit/1(Vector)
  Make Unit/1(Unit Vector) -> Multiply2/1
  vel/1 -> Multiply2/2  "vel"

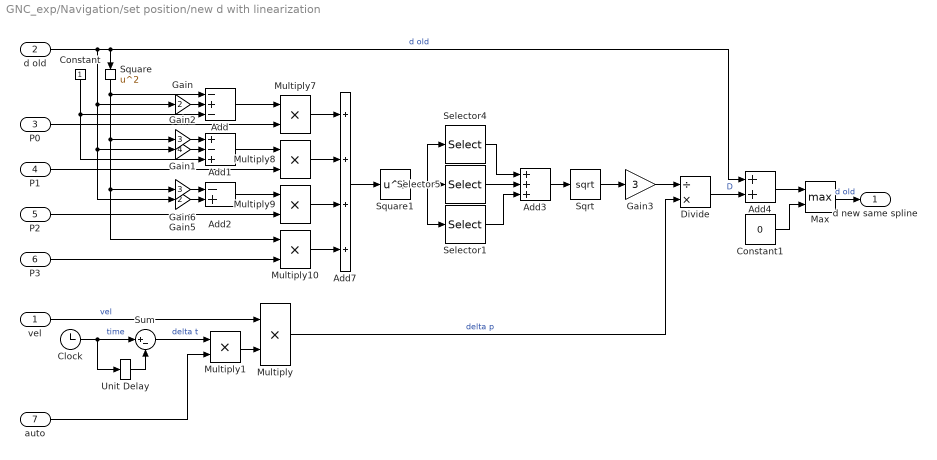
== system GNC_exp/Navigation/set position/new d with linearization ==
  vel : Inport
  d old : Inport  Port=2
  P0 : Inport  Port=3
  P1 : Inport  Port=4
  P2 : Inport  Port=5
  P3 : Inport  Port=6
  auto : Inport  Port=7
  Add : Sum  Inputs=-+-
  Add1 : Sum  Inputs=+-+
  Add2 : Sum  Inputs=-+
  Add3 : Sum  Inputs=+++
  Add4 : Sum
  Add7 : Sum  Inputs=++++
  Clock : Clock
  Constant : Constant
  Constant1 : Constant  Value=0
  Divide : Product  Inputs=/*
  Gain : Gain  Gain=2
  Gain1 : Gain  Gain=4
  Gain2 : Gain  Gain=3
  Gain3 : Gain  Gain=3
  Gain5 : Gain  Gain=2
  Gain6 : Gain  Gain=3
  Max : MinMax  Function=max  Inputs=2
  Multiply{,1,7..10} (6 alike) : Product
  Selector1 : Selector  IndexMode=Zero-based  InputPortWidth=3  IndexOptions=Index vector (dialog)  Indices=2  OutputSizes=1
  Selector4 : Selector  IndexMode=Zero-based  InputPortWidth=3  IndexOptions=Index vector (dialog)  Indices=0  OutputSizes=1
  Selector5 : Selector  IndexMode=Zero-based  InputPortWidth=3  IndexOptions=Index vector (dialog)  Indices=1  OutputSizes=1
  Sqrt : Sqrt  SaturateOnIntegerOverflow=on
  Square : Math  Operator=square  SaturateOnIntegerOverflow=on
  Square1 : Math  Operator=square  SaturateOnIntegerOverflow=on
  Sum : Sum  Inputs=|+-
  Unit Delay : UnitDelay  SampleTime=-1
  d new same spline : Outport
  wires:
  Add7/1 -> Square1/1
  Multiply8/1 -> Add7/2
  Multiply9/1 -> Add7/3
  Square/1 -> Multiply10/1, Gain6/1, Gain2/1, Add/1
  Gain/1 -> Add/2
  Constant/1 -> Add1/3, Add/3
  Gain2/1 -> Add1/1
  Gain1/1 -> Add1/2
  Gain6/1 -> Add2/1
  Gain5/1 -> Add2/2
  Multiply10/1 -> Add7/4
  Add2/1 -> Multiply9/1
  Add1/1 -> Multiply8/1
  Add/1 -> Multiply7/1
  Multiply7/1 -> Add7/1
  Selector5/1 -> Add3/2
  Gain3/1 -> Divide/1
  Divide/1 -> Add4/2  "D"
  Selector4/1 -> Add3/1
  Add3/1 -> Sqrt/1
  Square1/1 -> Selector1/1, Selector4/1, Selector5/1
  Sqrt/1 -> Gain3/1
  Selector1/1 -> Add3/3
  Add4/1 -> Max/1
  Constant1/1 -> Max/2
  P1/1 -> Multiply8/2
  P2/1 -> Multiply9/2
  P0/1 -> Multiply7/2
  Max/1 -> d new same spline/1  "d old"
  P3/1 -> Multiply10/2
  d old/1 -> Add4/1, Square/1, Gain/1, Gain5/1, Gain1/1  "d old"
  Multiply1/1 -> Multiply/2
  auto/1 -> Multiply1/2
  Clock/1 -> Unit Delay/1, Sum/1  "time"
  Multiply/1 -> Divide/2  "delta p"
  Unit Delay/1 -> Sum/2
  Sum/1 -> Multiply1/1  "delta t"
  vel/1 -> Multiply/1  "vel"

== system GNC_exp/Control/Create Path Frame/Make X Vector/Make Unit ==
  Vector : Inport
  Multiply : Product
  Reciprocal Sqrt : Sqrt  Operator=rSqrt  SaturateOnIntegerOverflow=on
  Square : Math  Operator=square  SaturateOnIntegerOverflow=on
  Sum of Elements : Sum  Inputs=+
  Unit Vector : Outport
  wires:
  Reciprocal Sqrt/1 -> Multiply/1
  Vector/1 -> Square/1, Multiply/2
  Square/1 -> Sum of Elements/1
  Multiply/1 -> Unit Vector/1
  Sum of Elements/1 -> Reciprocal Sqrt/1

== system GNC_exp/Control/Create Path Frame/Make Y Vector/Make Unit ==
  Vector : Inport
  Multiply : Product
  Reciprocal Sqrt : Sqrt  Operator=rSqrt  SaturateOnIntegerOverflow=on
  Square : Math  Operator=square  SaturateOnIntegerOverflow=on
  Sum of Elements : Sum  Inputs=+
  Unit Vector : Outport
  wires:
  Reciprocal Sqrt/1 -> Multiply/1
  Vector/1 -> Square/1, Multiply/2
  Square/1 -> Sum of Elements/1
  Multiply/1 -> Unit Vector/1
  Sum of Elements/1 -> Reciprocal Sqrt/1

== system GNC_exp/Control/Create Path Frame/Make Z Vector/Make Unit ==
  Vector : Inport
  Multiply : Product
  Reciprocal Sqrt : Sqrt  Operator=rSqrt  SaturateOnIntegerOverflow=on
  Square : Math  Operator=square  SaturateOnIntegerOverflow=on
  Sum of Elements : Sum  Inputs=+
  Unit Vector : Outport
  wires:
  Reciprocal Sqrt/1 -> Multiply/1
  Vector/1 -> Square/1, Multiply/2
  Square/1 -> Sum of Elements/1
  Multiply/1 -> Unit Vector/1
  Sum of Elements/1 -> Reciprocal Sqrt/1

== system GNC_exp/Navigation/calc v/Create Path Frame/Make X Vector ==
  Velocity Vector : Inport
  Make Unit : Subsystem
  Transpose : Math  Operator=transpose  SaturateOnIntegerOverflow=on
  X Vector : Outport
  wires:
  Velocity Vector/1 -> Make Unit/1(Vector)
  Make Unit/1(Unit Vector) -> Transpose/1
  Transpose/1 -> X Vector/1

== system GNC_exp/Navigation/calc v/Create Path Frame/Make Y Vector ==
  Velocity Vector : Inport
  Constant : Constant  Value=0
  Demux : Demux  Outputs=3
  Gain : Gain  Gain=-1
  Make Unit : Subsystem
  Matrix Concatenate : Concatenate  NumInputs=3  Mode=Multidimensional array
  Terminator : Terminator
  Y Vector : Outport
  wires:
  Make Unit/1(Unit Vector) -> Y Vector/1
  Velocity Vector/1 -> Demux/1
  Demux/3 -> Terminator/1
  Demux/2 -> Gain/1
  Gain/1 -> Matrix Concatenate/1
  Demux/1 -> Matrix Concatenate/2
  Constant/1 -> Matrix Concatenate/3
  Matrix Concatenate/1 -> Make Unit/1(Vector)

== system GNC_exp/Navigation/calc v/Create Path Frame/Make Z Vector ==
  Velocity Vector : Inport
  Add : Sum
  Demux : Demux  Outputs=3
  Gain : Gain  Gain=-1
  Gain1 : Gain  Gain=-1
  Make Unit : Subsystem
  Matrix Concatenate : Concatenate  NumInputs=3  Mode=Multidimensional array
  Multiply : Product
  Multiply1 : Product
  Square : Math  Operator=square  SaturateOnIntegerOverflow=on
  Square1 : Math  Operator=square  SaturateOnIntegerOverflow=on
  Z Vector : Outport
  wires:
  Make Unit/1(Unit Vector) -> Z Vector/1
  Velocity Vector/1 -> Demux/1
  Demux/3 -> Multiply/2, Multiply1/2
  Matrix Concatenate/1 -> Make Unit/1(Vector)
  Multiply/1 -> Gain/1
  Gain/1 -> Matrix Concatenate/1
  Demux/1 -> Square/1, Multiply/1
  Multiply1/1 -> Gain1/1
  Gain1/1 -> Matrix Concatenate/2
  Demux/2 -> Square1/1, Multiply1/1
  Add/1 -> Matrix Concatenate/3
  Square/1 -> Add/1
  Square1/1 -> Add/2

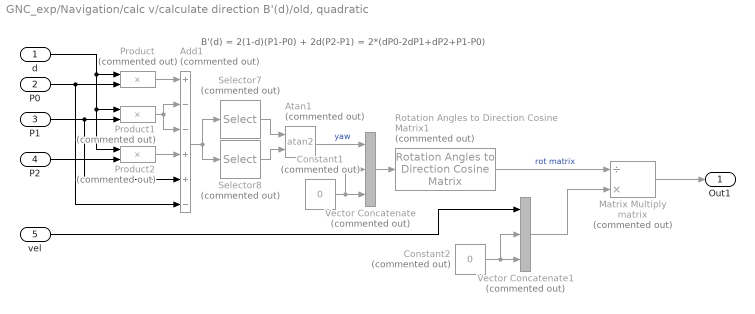
== system GNC_exp/Navigation/calc v/calculate direction B'(d)/old, quadratic ==
  note: B'(d) = 2(1-d)(P1-P0) + 2d(P2-P1) = 2*(dP0-2dP1+dP2+P1-P0)
  d : Inport
  P0 : Inport  Port=2
  P1 : Inport  Port=3
  P2 : Inport  Port=4
  vel : Inport  Port=5
  Add1 : Sum  Commented=on  Inputs=+--++-
  Atan1 : Trigonometry  Commented=on  Operator=atan2
  Constant1 : Constant  Commented=on  Value=0
  Constant2 : Constant  Commented=on  Value=0
  Matrix Multiply : Product  Commented=on  Inputs=/*  Multiplication=Matrix(*)
  Product : Product  Commented=on
  Product1 : Product  Commented=on
  Product2 : Product  Commented=on
  Rotation Angles to Direction Cosine Matrix1 : sharedtransform/Rotation Angles to Direction Cosine Matrix  Commented=on  rotationOrder=ZYX  aMode=aMode
      settings: SourceProductBaseCode=AE
  Selector7 : Selector  Commented=on  IndexMode=Zero-based  InputPortWidth=3  IndexOptions=Index vector (dialog)  Indices=1  OutputSizes=1
  Selector8 : Selector  Commented=on  IndexMode=Zero-based  InputPortWidth=3  IndexOptions=Index vector (dialog)  Indices=0  OutputSizes=1
  Vector Concatenate : Concatenate  Commented=on  NumInputs=3
  Vector Concatenate1 : Concatenate  Commented=on  NumInputs=3
  Out1 : Outport
  wires:
  Product2/1 -> Add1/4
  P1/1 -> Add1/5, Product1/2
  Rotation Angles to Direction Cosine Matrix1/1 -> Matrix Multiply/1  "rot matrix"
  P2/1 -> Product2/2
  Add1/1 -> Selector8/1, Selector7/1
  Product/1 -> Add1/1
  P0/1 -> Add1/6, Product/2
  d/1 -> Product2/1, Product1/1, Product/1
  Constant1/1 -> Vector Concatenate/2, Vector Concatenate/3
  Vector Concatenate1/1 -> Matrix Multiply/2
  Product1/1 -> Add1/3, Add1/2
  Vector Concatenate/1 -> Rotation Angles to Direction Cosine Matrix1/1
  Selector7/1 -> Atan1/1
  vel/1 -> Vector Concatenate1/1
  Constant2/1 -> Vector Concatenate1/2, Vector Concatenate1/3
  Matrix Multiply/1 -> Out1/1
  Selector8/1 -> Atan1/2
  Atan1/1 -> Vector Concatenate/1  "yaw"

== system GNC_exp/Navigation/calculate desired/calc pos B(d)/old, quadratic ==
  note: B(d) = (1-d)*u.*((1-d)*P0+d*P1)+d*u.*((1-d)*P1 + d*P2);
  d : Inport
  In2 : Inport  Port=2
  In3 : Inport  Port=3
  In4 : Inport  Port=4
  Add : Sum  Commented=on
  Add1 : Sum  Commented=on
  Add2 : Sum  Commented=on
  Constant : Constant  Commented=on
  Multiply{2..7} (6 alike) : Product  Commented=on
  Sum : Sum  Commented=on  Inputs=|+-
  Out1 : Outport
  wires:
  In4/1 -> Multiply5/1
  Constant/1 -> Sum/1
  Multiply7/1 -> Add2/2
  d/1 -> Multiply5/2, Multiply7/1, Multiply3/1, Sum/2
  Multiply3/1 -> Add/2
  Multiply5/1 -> Add1/2
  Multiply4/1 -> Add1/1
  Sum/1 -> Multiply4/2, Multiply6/2, Multiply2/1  "1-d"
  In3/1 -> Multiply4/1, Multiply3/2
  Multiply2/1 -> Add/1
  Add2/1 -> Out1/1
  Add1/1 -> Multiply7/2
  Multiply6/1 -> Add2/1
  In2/1 -> Multiply2/2
  Add/1 -> Multiply6/1

== system GNC_exp/Navigation/calculate desired/calculate direction B'(d)/Make Unit ==
  Vector : Inport
  Multiply : Product
  Reciprocal Sqrt : Sqrt  Operator=rSqrt  SaturateOnIntegerOverflow=on
  Square : Math  Operator=square  SaturateOnIntegerOverflow=on
  Sum of Elements : Sum  Inputs=+
  Transpose : Math  Operator=transpose  SaturateOnIntegerOverflow=on
  Unit Vector : Outport
  wires:
  Reciprocal Sqrt/1 -> Multiply/1
  Vector/1 -> Square/1, Multiply/2
  Square/1 -> Sum of Elements/1
  Multiply/1 -> Transpose/1
  Sum of Elements/1 -> Reciprocal Sqrt/1
  Transpose/1 -> Unit Vector/1
